simulink model "zad3_simulink"  (R2023b)
settings: Solver=VariableStepAuto  StartTime=0.0  StopTime=40  RelTol=1e-3
settings Model: Creator=micha  LastModifiedBy=micha

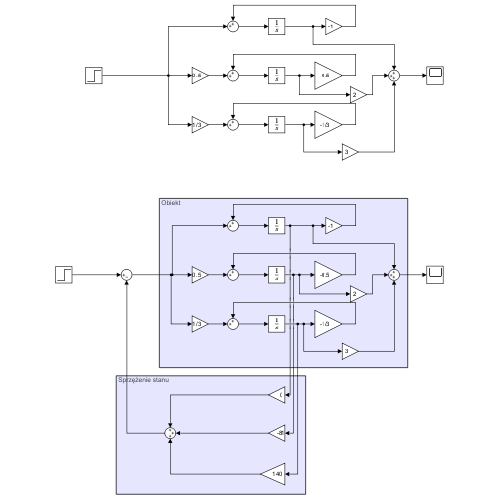
[thumbnail: Simulink's stored preview of the top-level diagram]
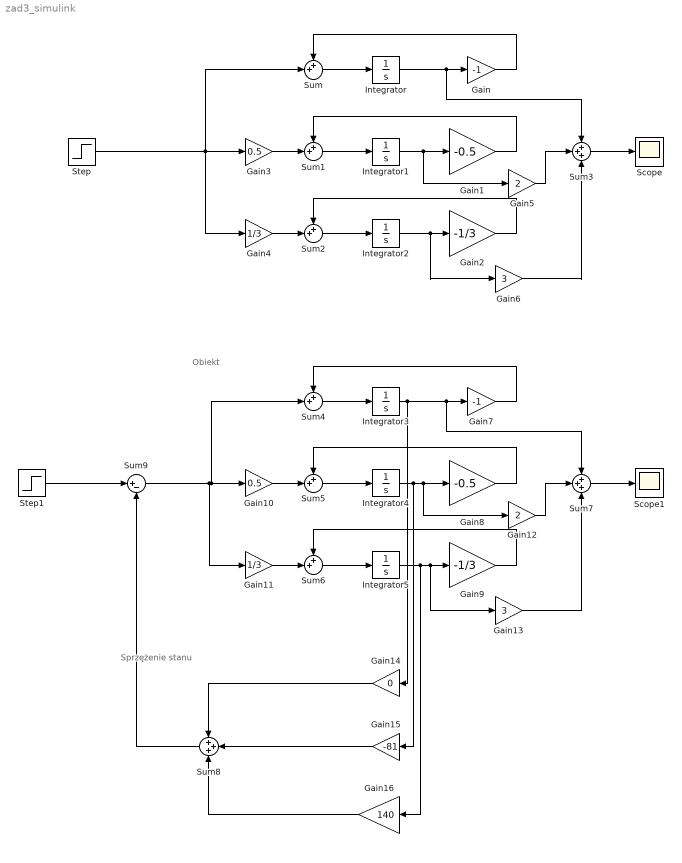
== system zad3_simulink ==
  note: Obiekt
  note: Sprzężenie stanu
  Gain : Gain  Gain=-1
  Gain1 : Gain  Gain=-0.5
  Gain10 : Gain  Gain=0.5
  Gain11 : Gain  Gain=1/3
  Gain12 : Gain  Gain=2
  Gain13 : Gain  Gain=3
  Gain14 : Gain  Gain=0
  Gain15 : Gain  Gain=-81
  Gain16 : Gain  Gain=140
  Gain2 : Gain  Gain=-1/3
  Gain3 : Gain  Gain=0.5
  Gain4 : Gain  Gain=1/3
  Gain5 : Gain  Gain=2
  Gain6 : Gain  Gain=3
  Gain7 : Gain  Gain=-1
  Gain8 : Gain  Gain=-0.5
  Gain9 : Gain  Gain=-1/3
  Integrator{,1..5} (6 alike) : Integrator
  Scope : Scope
  Scope1 : Scope
  Step : Step  SampleTime=0
  Step1 : Step  SampleTime=0
  Sum{,1..2,4..6} (6 alike) : Sum  Inputs=++|
  Sum3 : Sum  Inputs=+++
  Sum7 : Sum  Inputs=+++
  Sum8 : Sum  Inputs=+++
  Sum9 : Sum  Inputs=|+-
  wires:
  Integrator/1 -> Sum3/1, Gain/1
  Sum/1 -> Integrator/1
  Gain/1 -> Sum/1
  Gain1/1 -> Sum1/1
  Sum1/1 -> Integrator1/1
  Gain2/1 -> Sum2/1
  Sum2/1 -> Integrator2/1
  Gain4/1 -> Sum2/2
  Gain3/1 -> Sum1/2
  Step/1 -> Gain4/1, Sum/2, Gain3/1
  Integrator1/1 -> Gain5/1, Gain1/1
  Integrator2/1 -> Gain6/1, Gain2/1
  Sum3/1 -> Scope/1
  Gain5/1 -> Sum3/2
  Gain6/1 -> Sum3/3
  Sum7/1 -> Scope1/1
  Gain13/1 -> Sum7/3
  Integrator5/1 -> Gain16/1, Gain13/1, Gain9/1
  Sum6/1 -> Integrator5/1
  Gain9/1 -> Sum6/1
  Sum5/1 -> Integrator4/1
  Integrator4/1 -> Gain15/1, Gain12/1, Gain8/1
  Gain8/1 -> Sum5/1
  Gain7/1 -> Sum4/1
  Gain10/1 -> Sum5/2
  Gain11/1 -> Sum6/2
  Sum4/1 -> Integrator3/1
  Gain12/1 -> Sum7/2
  Integrator3/1 -> Gain14/1, Sum7/1, Gain7/1
  Gain14/1 -> Sum8/1
  Gain15/1 -> Sum8/2
  Gain16/1 -> Sum8/3
  Sum9/1 -> Gain11/1, Sum4/2, Gain10/1
  Step1/1 -> Sum9/1
  Sum8/1 -> Sum9/2
